simulink model "LTDKsimulation1"  (R2014a)
settings: Solver=ode45  StartTime=0.0  StopTime=10  RelTol=1e-3
settings Model: Creator=tri  LastModifiedBy=tri
settings DataIOCC: InspectSignalLogs=on

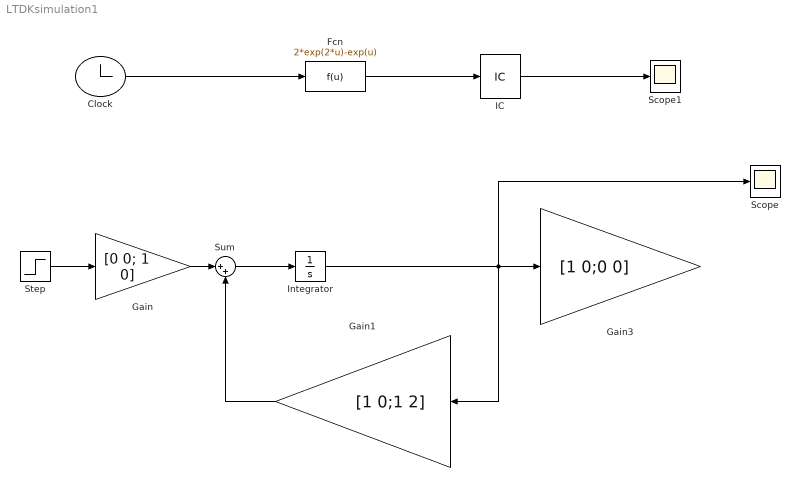
== system LTDKsimulation1 ==
  Clock : Clock
  Fcn : Fcn  Expr=2*exp(2*u)-exp(u)
  Gain : Gain  Gain=[0 0; 1 0]
  Gain1 : Gain  Gain=[1 0;1 2]
  Gain3 : Gain  Gain=[1 0;0 0]
  IC : InitialCondition  Value=0
  Integrator : Integrator
  Scope : Scope
  Scope1 : Scope
  Step : Step  SampleTime=0
  Sum : Sum  Inputs=|++
  wires:
  Gain/1 -> Sum/1
  Sum/1 -> Integrator/1
  Gain1/1 -> Sum/2
  Integrator/1 -> Scope/1, Gain3/1, Gain1/1
  Step/1 -> Gain/1
  Clock/1 -> Fcn/1
  Fcn/1 -> IC/1
  IC/1 -> Scope1/1
